simulink model "ACC_test_sim"  (R2023a)
settings: Solver=FixedStepAuto  StartTime=0.0  StopTime=100  FixedStep=0.001  RelTol=1e-3
values from neighbouring files (symbols this model uses):
  b = 50    [ACC_test.m]
  den = [m b]    [ACC_test.m]
  den_dc = [1 (1/J)*(D+KtRa*Kb)]    [ACC_test.m]
  m = 1000    [ACC_test.m]
  num = 1    [ACC_test.m]
  num_dc = KtRa/J    (= 4916.66666667)    [ACC_test.m]
undefined symbols (not defined in the file or in its folder): sigbuilder_block
libraries: slpidlib x10, simulink x6, simulink_extras x6, sim3dautolib x6, sim3dlib x3, mpclib x1
(part 1 of 2)
settings Model: Creator=joeri  LastModifiedBy=joeri
settings DataIOCC: ReturnWorkspaceOutputs=off
settings ModelReferenceCC: EnableRefExpFcnMdlSchedulingChecks=on

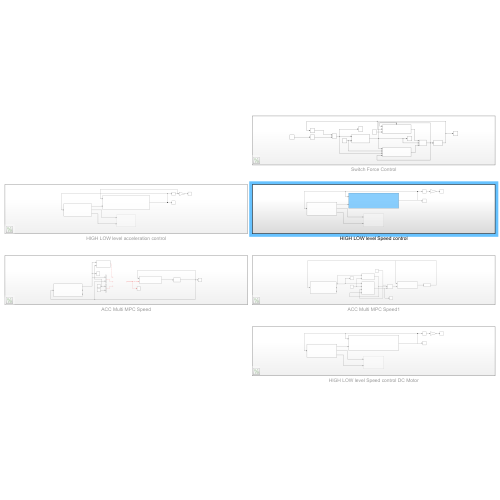
[thumbnail: Simulink's stored preview of the top-level diagram]
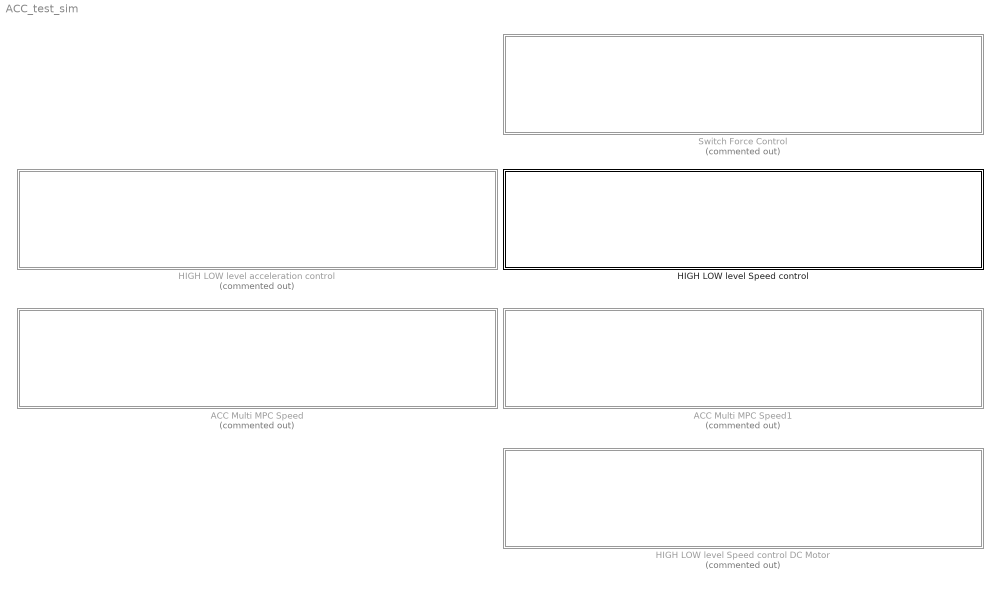
== system ACC_test_sim ==
  ACC Multi MPC Speed : Subsystem  Commented=on
  ACC Multi MPC Speed1 : Subsystem  Commented=on
  HIGH LOW level Speed control : Subsystem
  HIGH LOW level Speed control DC Motor : Subsystem  Commented=on
  HIGH LOW level acceleration control : Subsystem  Commented=on
  Switch Force Control : Subsystem  Commented=on

== system ACC_test_sim/ACC Multi MPC Speed ==
  Constant1 : Constant  Value=30/3.6
  Constant2 : Constant  Value=20
  Mux : Mux  Inputs=2
  Mux1 : Mux  Inputs=2
  Scope : Scope
  Scope1 : Scope
  Scope2 : Scope
  Sensors : Subsystem
  Speed Feedback Control : Subsystem
  Switcher : Subsystem
  Transfer Fcn (with initial outputs) : simulink_extras/Additional Linear/Transfer Fcn (with initial outputs)  N=num  D=den  Y0=30/3.6  U0=0
  wires:
  Transfer Fcn (with initial outputs)/1 -> Speed Feedback Control/1(Reference speed), Scope/1, Mux1/2, Sensors/1(MORE Vehicle speed)  "MORE Vehicle Speed"
  Speed Feedback Control/1(Control effort) -> Transfer Fcn (with initial outputs)/1
  ? -> Scope2/1, Speed Feedback Control/2(Speed)
  Sensors/1(Distance Gap) -> Switcher/1(Gap), Scope1/1, Mux1/1
  Constant1/1 -> Mux/2
  Constant2/1 -> Switcher/2(Desired Distance), Mux/1
  Mux/1 -> ?
  Mux1/1 -> ?
  Switcher/1(Output) -> ?

== system ACC_test_sim/ACC Multi MPC Speed1 ==
  Constant : Constant  Value=20
  MPC Speed : mpclib/MPC Controller  SCDEnableBlockLinearizationSpecification=on  mpcobj=mpc1  is_multiple=0  enable_value=0  return_u0=off  updateMPCinCallerWorkspace=on  md_inport=off  mv_inport=off  uref_inport=off  return_cost=off  return_mvseq=off  return_qpstatus=off  return_xseq=off  return_state=off  return_ovseq=off  state_inport=off  umin_inport=off  umax_inport=off  ymin_inport=off  ymax_inport=on  cc_inport=off  ywt_inport=off  uwt_inport=off  duwt_inport=off  rhoeps_inport=off  pm_inport=off  MaximumP=10  HorizonChoice=FixedHorizon  n_ts=0.1  n_p=30  n_mv=1  n_md=0  n_ud=0  n_mo=1  n_uo=0  BlockDataType=double  SampleTimeInherited=off  switch_inport=on
  Scope1 : Scope
  Scope2 : Scope
  Sensors : Subsystem
  Speed Feedback Control : Subsystem
  Switch : Switch  Criteria=u2 > Threshold  SaturateOnIntegerOverflow=off  InputSameDT=off
  Switcher : Subsystem
  Transfer Fcn (with initial outputs) : simulink_extras/Additional Linear/Transfer Fcn (with initial outputs)  N=num  D=den  Y0=30/3.6  U0=0
  v_d : Constant  Value=30/3.6
  wires:
  Transfer Fcn (with initial outputs)/1 -> Sensors/1(MORE Vehicle speed), Speed Feedback Control/1(Reference speed)  "MORE Vehicle Speed"
  Sensors/1(Distance Gap) -> Switcher/1(Gap), Scope1/1, MPC Speed/1
  Speed Feedback Control/1(Control effort) -> Transfer Fcn (with initial outputs)/1
  Constant/1 -> MPC Speed/2, Switcher/2(Desired Distance)
  Switch/1 -> Speed Feedback Control/2(Speed setpoint)
  MPC Speed/1 -> Scope2/1, Switch/3
  v_d/1 -> MPC Speed/3, Switch/1
  Switcher/1(Output) -> MPC Speed/4, Switch/2

== system ACC_test_sim/HIGH LOW level Speed control ==
  3D Sim : Subsystem  Commented=on
  Derivative : Derivative
  Model And Control : Subsystem
  Scope1 : Scope
  Scope2 : Scope
  Sensors : Subsystem
  m/s/s to G : Gain  Gain=1/9.81
  wires:
  Derivative/1 -> m/s/s to G/1
  m/s/s to G/1 -> Scope2/1
  Model And Control/1(MORE Vehicle Speed [m/s]) -> Scope1/1, Model And Control/1(Reference speed [m/s]), Sensors/1(MORE Vehicle speed), Derivative/1
  Sensors/1(Distance Gap) -> Model And Control/2(Distance Gap [m])
  Sensors/2(MORE Vehicle distance) -> 3D Sim/1(MORE Vehicle Distance)
  Sensors/3(Leading Vehicle distance) -> 3D Sim/2(Leading Vehicle distance)

== system ACC_test_sim/HIGH LOW level Speed control DC Motor ==
  3D Sim : Subsystem  Commented=on
  Derivative : Derivative
  Model And Control : Subsystem
  Scope1 : Scope
  Scope2 : Scope
  Sensors : Subsystem
  m/s/s to G : Gain  Gain=1/9.81
  wires:
  Derivative/1 -> m/s/s to G/1
  m/s/s to G/1 -> Scope2/1
  Model And Control/1(MORE Vehicle Speed) -> Scope1/1, Model And Control/1(Reference speed), Sensors/1(MORE Vehicle speed), Derivative/1
  Sensors/1(Distance Gap) -> Model And Control/2(Distance Gap)
  Sensors/2(MORE Vehicle distance) -> 3D Sim/1(MORE Vehicle Distance)
  Sensors/3(Leading Vehicle distance) -> 3D Sim/2(Leading Vehicle distance)

== system ACC_test_sim/HIGH LOW level acceleration control ==
  3D Sim : Subsystem  Commented=on
  Derivative : Derivative
  Model And Control : Subsystem
  Scope1 : Scope
  Scope2 : Scope
  Sensors : Subsystem
  m/s/s to G : Gain  Gain=1/9.81
  wires:
  Derivative/1 -> Model And Control/1(Reference acc.), m/s/s to G/1
  m/s/s to G/1 -> Scope2/1
  Model And Control/1(MORE Vehicle Speed) -> Scope1/1, Sensors/1(MORE Vehicle speed), Derivative/1
  Sensors/1(Distance Gap) -> Model And Control/2(Distance Gap)
  Sensors/2(MORE Vehicle distance) -> 3D Sim/1(MORE Vehicle Distance)
  Sensors/3(Leading Vehicle distance) -> 3D Sim/2(Leading Vehicle distance)

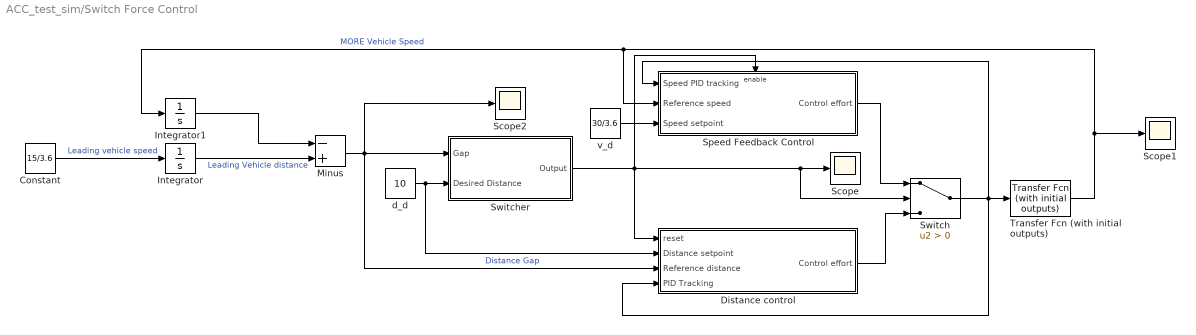
== system ACC_test_sim/Switch Force Control ==
  Constant : Constant  Value=15/3.6
  Distance control : Subsystem
  Integrator : Integrator  InitialCondition=100
  Integrator1 : Integrator
  Minus : Sum  Inputs=-+
  Scope : Scope
  Scope1 : Scope
  Scope2 : Scope
  Speed Feedback Control : Subsystem
  Switch : Switch  Criteria=u2 > Threshold  SaturateOnIntegerOverflow=off  InputSameDT=off
  Switcher : Subsystem
  Transfer Fcn (with initial outputs) : simulink_extras/Additional Linear/Transfer Fcn (with initial outputs)  N=num  D=den  Y0=30/3.6  U0=0
  d_d : Constant  Value=10
  v_d : Constant  Value=30/3.6
  wires:
  Minus/1 -> Switcher/1(Gap), Scope2/1, Distance control/3(Reference distance)  "Distance Gap"
  Distance control/1(Control effort) -> Switch/3
  Speed Feedback Control/1(Control effort) -> Switch/1
  Transfer Fcn (with initial outputs)/1 -> Speed Feedback Control/2(Reference speed), Integrator1/1, Scope1/1  "MORE Vehicle Speed"
  Switch/1 -> Speed Feedback Control/1(Speed PID tracking), Distance control/4(PID Tracking), Transfer Fcn (with initial outputs)/1
  Switcher/1(Output) -> Speed Feedback Control/Enable, Distance control/1(reset), Scope/1, Switch/2
  Integrator/1 -> Minus/2  "Leading Vehicle distance"
  v_d/1 -> Speed Feedback Control/3(Speed setpoint)
  d_d/1 -> Distance control/2(Distance setpoint), Switcher/2(Desired Distance)
  Integrator1/1 -> Minus/1
  Constant/1 -> Integrator/1  "Leading vehicle speed"

== system ACC_test_sim/ACC Multi MPC Speed/Sensors ==
  MORE Vehicle speed : Inport
  Constant : Constant  Value=20/3.6
  Integrator : Integrator  InitialCondition=100
  Integrator1 : Integrator
  Minus : Sum  Inputs=-+
  Minus1 : Sum  Inputs=+-
  Signal Builder : Subsystem  Tag=STV Subsys  LoadFcn=sigbuilder_block('load');  StartFcn=sigbuilder_block('start');  StopFcn=sigbuilder_block('stop');  ClipboardFcn=sigbuilder_block('clipboard');  mask(Sigbuilder block){tuvar=[0:10]}
      mask help: Simulink:masks:SigbuilderBlock_MD
      mask init:
      | if ~strcmp(get_param(bdroot(gcbh),'SimulationStatus'),'stopped') tuvar = sigbuilder_block('maskInit'); end
      settings: CopyFcn=sigbuilder_block('copy');  DeleteFcn=sigbuilder_block('delete');  ModelCloseFcn=sigbuilder_block('modelClose');  PreSaveFcn=sigbuilder_block('preSave');  PauseFcn=sigbuilder_block('pause');  ContinueFcn=sigbuilder_block('continue');  NameChangeFcn=sigbuilder_block('namechange');  OpenFcn=sigbuilder_block('open',[446.4 127.8 550.8 400.2 ]);  CloseFcn=sigbuilder_block('close');
      mask Display: plot(0, 0, 100, 100,[2, 2, 32, 32, 2], [68, 8, 8, 68, 68],[32, 2], [38, 38], [32, 19, 2],[53, 60, 44], [32, 17, 17, 2],[16, 16, 31, 31]);txt = getActiveGroup(gcbh);text(2, 100, txt,'verticalAlignment', 'top');
  Distance Gap : Outport
  MORE Vehicle distance : Outport  Port=2
  Relative speed : Outport  Port=3
  wires:
  Constant/1 -> Integrator/1, Minus1/2  "Leading vehicle speed"
  Minus1/1 -> Relative speed/1
  Minus/1 -> Distance Gap/1  "Distance Gap"
  Integrator1/1 -> MORE Vehicle distance/1, Minus/1
  MORE Vehicle speed/1 -> Integrator1/1, Minus1/1
  Integrator/1 -> Minus/2  "Leading Vehicle distance"

== system ACC_test_sim/ACC Multi MPC Speed/Speed Feedback Control ==
  Reference speed : Inport
  Speed : Inport  Port=2
  -5000 -5000 N1 : Saturate  UpperLimit=5000  LowerLimit=-5000
  Add : Sum
  Feed Forward : Subsystem
  PID Controller : slpidlib/PID Controller  Controller=PID  Form=Parallel  TimeDomain=Continuous-time  UseExternalTs=off  SampleTime=-1  IntegratorMethod=Forward Euler  FilterMethod=Forward Euler  ControllerParametersSource=internal  P=2000  I=50  UseKiTs=off  D=10  N=100  UseFilter=on  TunerSelectOption=Transfer Function Based (PID Tuner App)  InitialConditionSource=internal  InitialConditionForIntegrator=0  InitialConditionForFilter=0  DifferentiatorICPrevScaledInput=0  ExternalReset=none  TrackingMode=off  Kt=0  LimitOutput=on  SatLimitsSource=internal  UpperSaturationLimit=5000  LowerSaturationLimit=-5000  LinearizeAsGain=on  AntiWindupMode=clamping  Kb=1  POutMin=[]  POutMax=[]  IOutMin=[]  IOutMax=[]  DOutMin=[]  DOutMax=[]  NOutMin=[]  NOutMax=[]  SumOutMin=[]  SumOutMax=[]  SaturationOutMin=[]  SaturationOutMax=[]  PParamMin=[]  PParamMax=[]  IParamMin=[]  IParamMax=[]  DParamMin=[]  DParamMax=[]  NParamMin=[]  NParamMax=[]  KbParamMin=[]  KbParamMax=[]  KtParamMin=[]  KtParamMax=[]  KbOutMin=[]  KbOutMax=[]  KtOutMin=[]  KtOutMax=[]  IntegratorOutMin=[]  IntegratorOutMax=[]  FilterOutMin=[]  FilterOutMax=[]  SumI1OutMin=[]  SumI1OutMax=[]  SumI2OutMin=[]  SumI2OutMax=[]  SumI3OutMin=[]  SumI3OutMax=[]  SumI4OutMin=[]  SumI4OutMax=[]  SumDOutMin=[]  SumDOutMax=[]  DifferentiatorOutMin=[]  DifferentiatorOutMax=[]  FilterDiffOutCoefMin=[]  FilterDiffOutCoefMax=[]  ReciprocalOutMin=[]  ReciprocalOutMax=[]  SumDenOutMin=[]  SumDenOutMax=[]  SumNumOutMin=[]  SumNumOutMax=[]  DivideOutMin=[]  DivideOutMax=[]  UdiffTsProdOutMin=[]  UdiffTsProdOutMax=[]  NTsProdOutMin=[]  NTsProdOutMax=[]  UintegralTsProdOutMin=[]  UintegralTsProdOutMax=[]  UngainTsProdOutMin=[]  UngainTsProdOutMax=[]  IntegratorContinuousStateAttributes=''  IntegratorStateMustResolveToSignalObject=off  IntegratorRTWStateStorageClass=Auto  FilterContinuousStateAttributes=''  FilterStateMustResolveToSignalObject=off  FilterRTWStateStorageClass=Auto  ParallelPVariant=InternalParameters  IdealPVariant=Disabled  IVariant=InternalParameters  DVariant=InternalParameters  IntegratorVariant=Continuous  SatVariant=Enabled  AWVariant=ContClampingParallel  PCopyVariant=Disabled  TRVariant=Disabled  FdbkBlocksVariant=Forward  IdealPFdbkVariant=Disabled  SatFdbkVariant=Disabled  DerivativeFilterVariant=ContFilter  NVariant=InternalParameters  NCopyVariant=Disabled  FilterICVariant=InternalICsFilter  IntegratorICVariant=InternalICs  ExternalResetVariant=Disabled  TRSumVariant=Passthrough  SumFdbkVariant=Disabled  SumVariant=Sum_PID  TsampFilterVariant=InternalTs  TsampNgainVariant=Passthrough  TsampIntegralVariant=Passthrough  ExternalSaturationOutDataTypeStr=Inherit: Same as second input  aMode=0
  Scope : Scope  NumInputPorts=3
  Sum1 : Sum  Inputs=|+-
  Control effort : Outport
  wires:
  Feed Forward/1(Out1) -> Add/1
  Reference speed/1 -> Sum1/2
  PID Controller/1 -> Add/2, Scope/2  "Controller Output, Force"
  Add/1 -> -5000 -5000 N1/1
  -5000 -5000 N1/1 -> Scope/3, Control effort/1  "Force"
  Speed/1 -> Sum1/1, Feed Forward/1(desired speed1), Scope/1
  Sum1/1 -> PID Controller/1  "E"

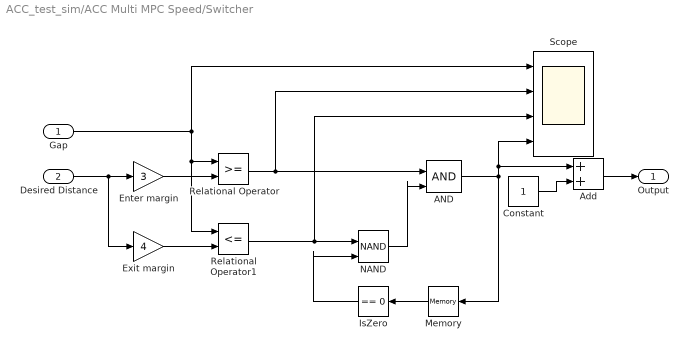
== system ACC_test_sim/ACC Multi MPC Speed/Switcher ==
  Gap : Inport
  Desired Distance : Inport  Port=2
  AND : Logic  IconShape=distinctive  AllPortsSameDT=off  OutDataTypeStr=boolean
  Add : Sum
  Constant : Constant
  Enter margin : Gain  Gain=3
  Exit margin : Gain  Gain=4
  IsZero : simulink/Logic and Bit Operations/Compare To Zero  relop===  OutDataTypeStr=boolean
  Memory : Memory
  NAND : Logic  Operator=NAND  IconShape=distinctive  AllPortsSameDT=off  OutDataTypeStr=boolean
  Relational Operator : RelationalOperator  OutDataTypeStr=boolean  RndMeth=Simplest  InputSameDT=off
  Relational Operator1 : RelationalOperator  Operator=<=  OutDataTypeStr=boolean  RndMeth=Simplest  InputSameDT=off
  Scope : Scope  NumInputPorts=4
  Output : Outport
  wires:
  Enter margin/1 -> Relational Operator/2
  Desired Distance/1 -> Exit margin/1, Enter margin/1
  Exit margin/1 -> Relational Operator1/2
  Relational Operator/1 -> AND/1, Scope/2
  Relational Operator1/1 -> NAND/1, Scope/3
  Memory/1 -> IsZero/1
  NAND/1 -> AND/2
  AND/1 -> Add/1, Scope/4, Memory/1
  IsZero/1 -> NAND/2
  Gap/1 -> Scope/1, Relational Operator1/1, Relational Operator/1
  Add/1 -> Output/1
  Constant/1 -> Add/2

== system ACC_test_sim/ACC Multi MPC Speed1/Sensors ==
  MORE Vehicle speed : Inport
  Constant : Constant  Value=20/3.6
  Integrator : Integrator  InitialCondition=100
  Integrator1 : Integrator
  Minus : Sum  Inputs=-+
  Signal Builder : Subsystem  Tag=STV Subsys  LoadFcn=sigbuilder_block('load');  StartFcn=sigbuilder_block('start');  StopFcn=sigbuilder_block('stop');  ClipboardFcn=sigbuilder_block('clipboard');  mask(Sigbuilder block){tuvar=[0:10]}
      mask help: Simulink:masks:SigbuilderBlock_MD
      mask init:
      | if ~strcmp(get_param(bdroot(gcbh),'SimulationStatus'),'stopped') tuvar = sigbuilder_block('maskInit'); end
      settings: CopyFcn=sigbuilder_block('copy');  DeleteFcn=sigbuilder_block('delete');  ModelCloseFcn=sigbuilder_block('modelClose');  PreSaveFcn=sigbuilder_block('preSave');  PauseFcn=sigbuilder_block('pause');  ContinueFcn=sigbuilder_block('continue');  NameChangeFcn=sigbuilder_block('namechange');  OpenFcn=sigbuilder_block('open',[446.4 127.8 550.8 400.2 ]);  CloseFcn=sigbuilder_block('close');
      mask Display: plot(0, 0, 100, 100,[2, 2, 32, 32, 2], [68, 8, 8, 68, 68],[32, 2], [38, 38], [32, 19, 2],[53, 60, 44], [32, 17, 17, 2],[16, 16, 31, 31]);txt = getActiveGroup(gcbh);text(2, 100, txt,'verticalAlignment', 'top');
  Distance Gap : Outport
  MORE Vehicle distance : Outport  Port=2
  Leading Vehicle distance : Outport  Port=3
  wires:
  Integrator/1 -> Leading Vehicle distance/1, Minus/2  "Leading Vehicle distance"
  MORE Vehicle speed/1 -> Integrator1/1
  Integrator1/1 -> Minus/1, MORE Vehicle distance/1
  Minus/1 -> Distance Gap/1  "Distance Gap"
  Signal Builder/1(Signal 1) -> Integrator/1

== system ACC_test_sim/ACC Multi MPC Speed1/Speed Feedback Control ==
  Reference speed : Inport
  Speed setpoint : Inport  Port=2
  -5000 -5000 N1 : Saturate  UpperLimit=5000  LowerLimit=-5000
  Add : Sum
  Feed Forward : Subsystem
  PID Controller : slpidlib/PID Controller  Controller=PID  Form=Parallel  TimeDomain=Continuous-time  UseExternalTs=off  SampleTime=-1  IntegratorMethod=Forward Euler  FilterMethod=Forward Euler  ControllerParametersSource=internal  P=2000  I=50  UseKiTs=off  D=10  N=100  UseFilter=on  TunerSelectOption=Transfer Function Based (PID Tuner App)  InitialConditionSource=internal  InitialConditionForIntegrator=0  InitialConditionForFilter=0  DifferentiatorICPrevScaledInput=0  ExternalReset=none  TrackingMode=off  Kt=0  LimitOutput=on  SatLimitsSource=internal  UpperSaturationLimit=5000  LowerSaturationLimit=-5000  LinearizeAsGain=on  AntiWindupMode=clamping  Kb=1  POutMin=[]  POutMax=[]  IOutMin=[]  IOutMax=[]  DOutMin=[]  DOutMax=[]  NOutMin=[]  NOutMax=[]  SumOutMin=[]  SumOutMax=[]  SaturationOutMin=[]  SaturationOutMax=[]  PParamMin=[]  PParamMax=[]  IParamMin=[]  IParamMax=[]  DParamMin=[]  DParamMax=[]  NParamMin=[]  NParamMax=[]  KbParamMin=[]  KbParamMax=[]  KtParamMin=[]  KtParamMax=[]  KbOutMin=[]  KbOutMax=[]  KtOutMin=[]  KtOutMax=[]  IntegratorOutMin=[]  IntegratorOutMax=[]  FilterOutMin=[]  FilterOutMax=[]  SumI1OutMin=[]  SumI1OutMax=[]  SumI2OutMin=[]  SumI2OutMax=[]  SumI3OutMin=[]  SumI3OutMax=[]  SumI4OutMin=[]  SumI4OutMax=[]  SumDOutMin=[]  SumDOutMax=[]  DifferentiatorOutMin=[]  DifferentiatorOutMax=[]  FilterDiffOutCoefMin=[]  FilterDiffOutCoefMax=[]  ReciprocalOutMin=[]  ReciprocalOutMax=[]  SumDenOutMin=[]  SumDenOutMax=[]  SumNumOutMin=[]  SumNumOutMax=[]  DivideOutMin=[]  DivideOutMax=[]  UdiffTsProdOutMin=[]  UdiffTsProdOutMax=[]  NTsProdOutMin=[]  NTsProdOutMax=[]  UintegralTsProdOutMin=[]  UintegralTsProdOutMax=[]  UngainTsProdOutMin=[]  UngainTsProdOutMax=[]  IntegratorContinuousStateAttributes=''  IntegratorStateMustResolveToSignalObject=off  IntegratorRTWStateStorageClass=Auto  FilterContinuousStateAttributes=''  FilterStateMustResolveToSignalObject=off  FilterRTWStateStorageClass=Auto  ParallelPVariant=InternalParameters  IdealPVariant=Disabled  IVariant=InternalParameters  DVariant=InternalParameters  IntegratorVariant=Continuous  SatVariant=Enabled  AWVariant=ContClampingParallel  PCopyVariant=Disabled  TRVariant=Disabled  FdbkBlocksVariant=Forward  IdealPFdbkVariant=Disabled  SatFdbkVariant=Disabled  DerivativeFilterVariant=ContFilter  NVariant=InternalParameters  NCopyVariant=Disabled  FilterICVariant=InternalICsFilter  IntegratorICVariant=InternalICs  ExternalResetVariant=Disabled  TRSumVariant=Passthrough  SumFdbkVariant=Disabled  SumVariant=Sum_PID  TsampFilterVariant=InternalTs  TsampNgainVariant=Passthrough  TsampIntegralVariant=Passthrough  ExternalSaturationOutDataTypeStr=Inherit: Same as second input  aMode=0
  Scope : Scope  NumInputPorts=3
  Sum1 : Sum  Inputs=|+-
  Control effort : Outport
  wires:
  Sum1/1 -> PID Controller/1  "E"
  Speed setpoint/1 -> Feed Forward/1(desired speed1), Sum1/1
  -5000 -5000 N1/1 -> Control effort/1, Scope/3  "Force"
  Add/1 -> -5000 -5000 N1/1
  Feed Forward/1(Out1) -> Scope/1, Add/1
  PID Controller/1 -> Scope/2, Add/2  "Controller Output, Force"
  Reference speed/1 -> Sum1/2

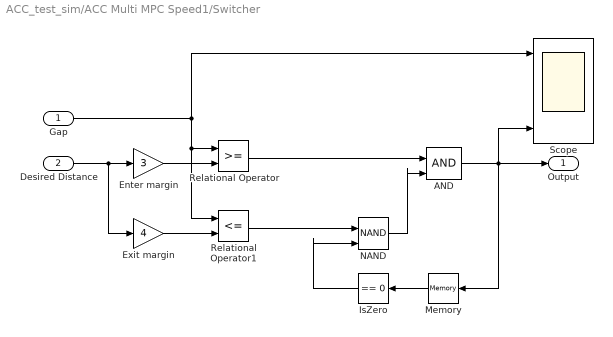
== system ACC_test_sim/ACC Multi MPC Speed1/Switcher ==
  Gap : Inport
  Desired Distance : Inport  Port=2
  AND : Logic  IconShape=distinctive  AllPortsSameDT=off  OutDataTypeStr=boolean
  Enter margin : Gain  Gain=3
  Exit margin : Gain  Gain=4
  IsZero : simulink/Logic and Bit Operations/Compare To Zero  relop===  OutDataTypeStr=boolean
  Memory : Memory
  NAND : Logic  Operator=NAND  IconShape=distinctive  AllPortsSameDT=off  OutDataTypeStr=boolean
  Relational Operator : RelationalOperator  OutDataTypeStr=boolean  RndMeth=Simplest  InputSameDT=off
  Relational Operator1 : RelationalOperator  Operator=<=  OutDataTypeStr=boolean  RndMeth=Simplest  InputSameDT=off
  Scope : Scope  NumInputPorts=4
  Output : Outport
  wires:
  Enter margin/1 -> Relational Operator/2
  Desired Distance/1 -> Exit margin/1, Enter margin/1
  Exit margin/1 -> Relational Operator1/2
  Relational Operator/1 -> AND/1
  Relational Operator1/1 -> NAND/1
  Memory/1 -> IsZero/1
  NAND/1 -> AND/2
  AND/1 -> Scope/4, Memory/1, Output/1
  IsZero/1 -> NAND/2
  Gap/1 -> Scope/1, Relational Operator1/1, Relational Operator/1

== system ACC_test_sim/HIGH LOW level Speed control/3D Sim ==
  MORE Vehicle Distance : Inport
  Leading Vehicle distance : Inport  Port=2
  Constant1 : Constant  Value=0
  Constant2 : Constant  Value=0
  Simulation 3D Scene Configuration : sim3dlib/Simulation 3D Scene Configuration  Priority=0  ProjectFormat=Default Scenes  SceneDesc=Straight road  ProjectName=C:\Program Files\MATLAB\R2022a\toolbox\shared\sim3d_projects\automotive_project\UE4\WindowsNoEditor\VehicleSimulation.exe  ScenePath=/Game/Maps/HwStrght  vehTagList={'Lead';'MORE';'Scene Origin'}  vehTag=MORE  OpVisEn=off  Ts=0.1  EnableWindow=on  EnableRemoteAccess=off  EnableWeather=off  SunAltitude=40.0  SunAzimuth=90  clouds=10  wind=1  fog=0  rain=0  sensorTag=MainCamera1  sensorId=1  sensorName=MainCamera1  mountLoc=Origin  offsetFlag=off  tmountOffset=[0, 0, 0]  rmountOffset=[0, 0, 0]  HorizontalResolution=1280  VerticalResolution=720  HorizontalFOV=60  mountPoint=[0 0 0]  mountOrientation=[0 0 0]  aMode=3  ID=1
  Simulation 3D Vehicle with Ground Following : sim3dautolib/Simulation 3D Vehicle with Ground Following  Priority=-1  PassVehMesh=Muscle car  MeshPath=/MathWorksSimulation/Vehicles/Muscle/Meshes/SK_MuscleCar.SK_MuscleCar  TrackWidth=1.9  WheelBase=3  WheelRadius=0.35  VehColor=Red  InitialPos=[0, 0, 0]  InitialRot=[0, 0, 0]  ActorName=Lead  SampleTime=-1  ActorType=SimulinkVehicle  ID=C  aMode=3  ActorTag=Lead  CoordinateScheme=ISO  VehLightsControl=off  HeadlightColor=[ 1, 1, 1 ]  HighBeamIntensity=100000  LowBeamIntensity=60000  HighBeamConeAngle=70  LowBeamConeAngle=70  LeftHeadlightOrientation=[ 0, 0 ]  RightHeadlightOrientation=[ 0, 0 ]  BrakelightIntensity=500  ReverselightIntensity=500  SignallightIntensity=500  SignallightPeriod=1  SignalPulseWidth=50  TransformOutportEnabled=off
  Simulation 3D Vehicle with Ground Following1 : sim3dautolib/Simulation 3D Vehicle with Ground Following  Priority=-1  PassVehMesh=Muscle car  MeshPath=/MathWorksSimulation/Vehicles/Muscle/Meshes/SK_MuscleCar.SK_MuscleCar  TrackWidth=1.9  WheelBase=3  WheelRadius=0.35  VehColor=Red  InitialPos=[0, 0, 0]  InitialRot=[0, 0, 0]  ActorName=MORE  SampleTime=-1  ActorType=SimulinkVehicle  ID=C  aMode=3  ActorTag=MORE  CoordinateScheme=ISO  VehLightsControl=off  HeadlightColor=[ 1, 1, 1 ]  HighBeamIntensity=100000  LowBeamIntensity=60000  HighBeamConeAngle=70  LowBeamConeAngle=70  LeftHeadlightOrientation=[ 0, 0 ]  RightHeadlightOrientation=[ 0, 0 ]  BrakelightIntensity=500  ReverselightIntensity=500  SignallightIntensity=500  SignallightPeriod=1  SignalPulseWidth=50  TransformOutportEnabled=off
  wires:
  Constant1/1 -> Simulation 3D Vehicle with Ground Following1/2, Simulation 3D Vehicle with Ground Following/2
  Constant2/1 -> Simulation 3D Vehicle with Ground Following/3, Simulation 3D Vehicle with Ground Following1/3
  MORE Vehicle Distance/1 -> Simulation 3D Vehicle with Ground Following1/1
  Leading Vehicle distance/1 -> Simulation 3D Vehicle with Ground Following/1

== system ACC_test_sim/HIGH LOW level Speed control/Model And Control ==
  Reference speed [m/s] : Inport
  Distance Gap [m] : Inport  Port=2
  ACC Distance Control : Subsystem
  CC Speed Feedback Control : Subsystem
  Desired Distance [m] : Constant  Value=20
  Desired Speed [m/s] : Constant  Value=10/3.6
  MORE Vehicle Transfer Function : simulink_extras/Additional Linear/Transfer Fcn (with initial outputs)  N=num  D=den  Y0=30/3.6  U0=0
  Switch : Switch  Criteria=u2 > Threshold  SaturateOnIntegerOverflow=off  InputSameDT=off
  Switcher : Subsystem
  To Workspace : ToWorkspace  VariableName=gap  SampleTime=-1
      settings: Save2DSignal=2-D array (concatenate along first dimension)
  MORE Vehicle Speed [m/s] : Outport
  wires:
  Desired Speed [m/s]/1 -> Switch/1, ACC Distance Control/1(Upper limit)
  Switcher/1(CC to ACC switch) -> Switch/2
  MORE Vehicle Transfer Function/1 -> MORE Vehicle Speed [m/s]/1  "MORE Vehicle Speed"
  ACC Distance Control/1(Speed Setpoint) -> Switch/3
  Distance Gap [m]/1 -> Switcher/1(Gap), To Workspace/1, ACC Distance Control/3(Distance gap)
  CC Speed Feedback Control/1(Control Effort [N]) -> MORE Vehicle Transfer Function/1
  Switch/1 -> ACC Distance Control/4(PID Tracking), CC Speed Feedback Control/2(Speed setpoint [m/s])
  Desired Distance [m]/1 -> ACC Distance Control/2(Distance setpoint), Switcher/2(Desired Distance)
  Reference speed [m/s]/1 -> CC Speed Feedback Control/1(Reference speed [m/s])

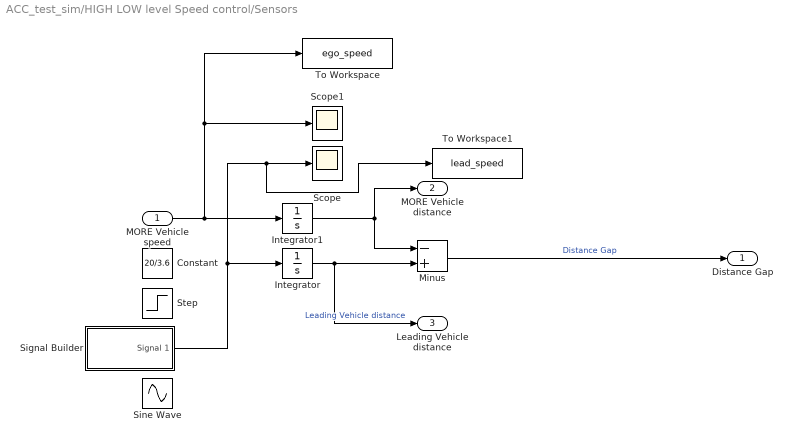
== system ACC_test_sim/HIGH LOW level Speed control/Sensors ==
  MORE Vehicle speed : Inport
  Constant : Constant  Value=20/3.6
  Integrator : Integrator  InitialCondition=100
  Integrator1 : Integrator
  Minus : Sum  Inputs=-+
  Scope : Scope
  Scope1 : Scope
  Signal Builder : Subsystem  Tag=STV Subsys  LoadFcn=sigbuilder_block('load');  StartFcn=sigbuilder_block('start');  StopFcn=sigbuilder_block('stop');  ClipboardFcn=sigbuilder_block('clipboard');  mask(Sigbuilder block){tuvar=[0:10]}
      mask help: Simulink:masks:SigbuilderBlock_MD
      mask init:
      | if ~strcmp(get_param(bdroot(gcbh),'SimulationStatus'),'stopped') tuvar = sigbuilder_block('maskInit'); end
      settings: CopyFcn=sigbuilder_block('copy');  DeleteFcn=sigbuilder_block('delete');  ModelCloseFcn=sigbuilder_block('modelClose');  PreSaveFcn=sigbuilder_block('preSave');  PauseFcn=sigbuilder_block('pause');  ContinueFcn=sigbuilder_block('continue');  NameChangeFcn=sigbuilder_block('namechange');  OpenFcn=sigbuilder_block('open',[446.4 127.8 550.8 400.2 ]);  CloseFcn=sigbuilder_block('close');
      mask Display: plot(0, 0, 100, 100,[2, 2, 32, 32, 2], [68, 8, 8, 68, 68],[32, 2], [38, 38], [32, 19, 2],[53, 60, 44], [32, 17, 17, 2],[16, 16, 31, 31]);txt = getActiveGroup(gcbh);text(2, 100, txt,'verticalAlignment', 'top');
  Sine Wave : Sin  Amplitude=3  Bias=15/3.6  Frequency=0.3  SampleTime=0
  Step : Step  Time=70  Before=20/3.6  After=10/3.6  SampleTime=0
  To Workspace : ToWorkspace  VariableName=ego_speed  SampleTime=-1
      settings: Save2DSignal=2-D array (concatenate along first dimension)
  To Workspace1 : ToWorkspace  VariableName=lead_speed  SampleTime=-1
      settings: Save2DSignal=2-D array (concatenate along first dimension)
  Distance Gap : Outport
  MORE Vehicle distance : Outport  Port=2
  Leading Vehicle distance : Outport  Port=3
  wires:
  Integrator/1 -> Leading Vehicle distance/1, Minus/2  "Leading Vehicle distance"
  MORE Vehicle speed/1 -> To Workspace/1, Scope1/1, Integrator1/1
  Integrator1/1 -> Minus/1, MORE Vehicle distance/1
  Minus/1 -> Distance Gap/1  "Distance Gap"
  Signal Builder/1(Signal 1) -> To Workspace1/1, Scope/1, Integrator/1

== system ACC_test_sim/HIGH LOW level Speed control DC Motor/3D Sim ==
  MORE Vehicle Distance : Inport
  Leading Vehicle distance : Inport  Port=2
  Constant1 : Constant  Value=0
  Constant2 : Constant  Value=0
  Simulation 3D Scene Configuration : sim3dlib/Simulation 3D Scene Configuration  Priority=0  ProjectFormat=Default Scenes  SceneDesc=Straight road  ProjectName=C:\Program Files\MATLAB\R2022a\toolbox\shared\sim3d_projects\automotive_project\UE4\WindowsNoEditor\VehicleSimulation.exe  ScenePath=/Game/Maps/HwStrght  vehTagList={'Lead';'MORE';'Scene Origin'}  vehTag=MORE  OpVisEn=off  Ts=0.1  EnableWindow=on  EnableRemoteAccess=off  EnableWeather=off  SunAltitude=40.0  SunAzimuth=90  clouds=10  wind=1  fog=0  rain=0  sensorTag=MainCamera1  sensorId=1  sensorName=MainCamera1  mountLoc=Origin  offsetFlag=off  tmountOffset=[0, 0, 0]  rmountOffset=[0, 0, 0]  HorizontalResolution=1280  VerticalResolution=720  HorizontalFOV=60  mountPoint=[0 0 0]  mountOrientation=[0 0 0]  aMode=3  ID=1
  Simulation 3D Vehicle with Ground Following : sim3dautolib/Simulation 3D Vehicle with Ground Following  Priority=-1  PassVehMesh=Muscle car  MeshPath=/MathWorksSimulation/Vehicles/Muscle/Meshes/SK_MuscleCar.SK_MuscleCar  TrackWidth=1.9  WheelBase=3  WheelRadius=0.35  VehColor=Red  InitialPos=[0, 0, 0]  InitialRot=[0, 0, 0]  ActorName=Lead  SampleTime=-1  ActorType=SimulinkVehicle  ID=C  aMode=3  ActorTag=Lead  CoordinateScheme=ISO  VehLightsControl=off  HeadlightColor=[ 1, 1, 1 ]  HighBeamIntensity=100000  LowBeamIntensity=60000  HighBeamConeAngle=70  LowBeamConeAngle=70  LeftHeadlightOrientation=[ 0, 0 ]  RightHeadlightOrientation=[ 0, 0 ]  BrakelightIntensity=500  ReverselightIntensity=500  SignallightIntensity=500  SignallightPeriod=1  SignalPulseWidth=50  TransformOutportEnabled=off
  Simulation 3D Vehicle with Ground Following1 : sim3dautolib/Simulation 3D Vehicle with Ground Following  Priority=-1  PassVehMesh=Muscle car  MeshPath=/MathWorksSimulation/Vehicles/Muscle/Meshes/SK_MuscleCar.SK_MuscleCar  TrackWidth=1.9  WheelBase=3  WheelRadius=0.35  VehColor=Red  InitialPos=[0, 0, 0]  InitialRot=[0, 0, 0]  ActorName=MORE  SampleTime=-1  ActorType=SimulinkVehicle  ID=C  aMode=3  ActorTag=MORE  CoordinateScheme=ISO  VehLightsControl=off  HeadlightColor=[ 1, 1, 1 ]  HighBeamIntensity=100000  LowBeamIntensity=60000  HighBeamConeAngle=70  LowBeamConeAngle=70  LeftHeadlightOrientation=[ 0, 0 ]  RightHeadlightOrientation=[ 0, 0 ]  BrakelightIntensity=500  ReverselightIntensity=500  SignallightIntensity=500  SignallightPeriod=1  SignalPulseWidth=50  TransformOutportEnabled=off
  wires:
  Constant1/1 -> Simulation 3D Vehicle with Ground Following1/2, Simulation 3D Vehicle with Ground Following/2
  Constant2/1 -> Simulation 3D Vehicle with Ground Following/3, Simulation 3D Vehicle with Ground Following1/3
  MORE Vehicle Distance/1 -> Simulation 3D Vehicle with Ground Following1/1
  Leading Vehicle distance/1 -> Simulation 3D Vehicle with Ground Following/1

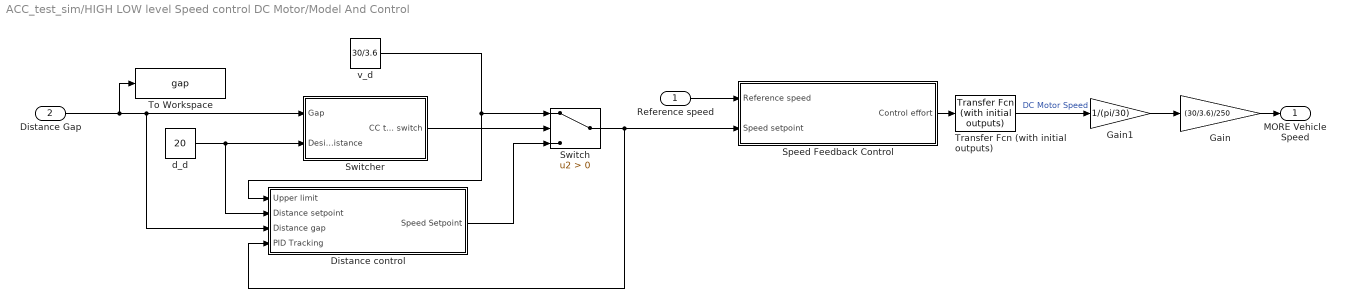
== system ACC_test_sim/HIGH LOW level Speed control DC Motor/Model And Control ==
  Reference speed : Inport
  Distance Gap : Inport  Port=2
  Distance control : Subsystem
  Gain : Gain  Gain=(30/3.6)/250
  Gain1 : Gain  Gain=1/(pi/30)
  Speed Feedback Control : Subsystem
  Switch : Switch  Criteria=u2 > Threshold  SaturateOnIntegerOverflow=off  InputSameDT=off
  Switcher : Subsystem
  To Workspace : ToWorkspace  VariableName=gap  SampleTime=-1
      settings: Save2DSignal=2-D array (concatenate along first dimension)
  Transfer Fcn (with initial outputs) : simulink_extras/Additional Linear/Transfer Fcn (with initial outputs)  N=num_dc  D=den_dc  Y0=250/(pi/30)  U0=0
  d_d : Constant  Value=20
  v_d : Constant  Value=30/3.6
  MORE Vehicle Speed : Outport
  wires:
  v_d/1 -> Switch/1, Distance control/1(Upper limit)
  Switcher/1(CC to ACC switch) -> Switch/2
  Transfer Fcn (with initial outputs)/1 -> Gain1/1  "DC Motor Speed"
  Distance control/1(Speed Setpoint) -> Switch/3
  Distance Gap/1 -> To Workspace/1, Switcher/1(Gap), Distance control/3(Distance gap)
  Speed Feedback Control/1(Control effort) -> Transfer Fcn (with initial outputs)/1
  Switch/1 -> Distance control/4(PID Tracking), Speed Feedback Control/2(Speed setpoint)
  d_d/1 -> Distance control/2(Distance setpoint), Switcher/2(Desired Distance)
  Reference speed/1 -> Speed Feedback Control/1(Reference speed)
  Gain/1 -> MORE Vehicle Speed/1
  Gain1/1 -> Gain/1

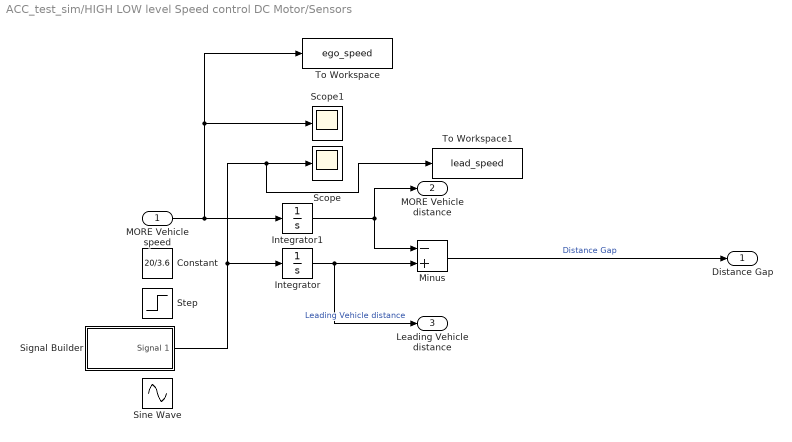
== system ACC_test_sim/HIGH LOW level Speed control DC Motor/Sensors ==
  MORE Vehicle speed : Inport
  Constant : Constant  Value=20/3.6
  Integrator : Integrator  InitialCondition=100
  Integrator1 : Integrator
  Minus : Sum  Inputs=-+
  Scope : Scope
  Scope1 : Scope
  Signal Builder : Subsystem  Tag=STV Subsys  LoadFcn=sigbuilder_block('load');  StartFcn=sigbuilder_block('start');  StopFcn=sigbuilder_block('stop');  ClipboardFcn=sigbuilder_block('clipboard');  mask(Sigbuilder block){tuvar=[0:10]}
      mask help: Simulink:masks:SigbuilderBlock_MD
      mask init:
      | if ~strcmp(get_param(bdroot(gcbh),'SimulationStatus'),'stopped') tuvar = sigbuilder_block('maskInit'); end
      settings: CopyFcn=sigbuilder_block('copy');  DeleteFcn=sigbuilder_block('delete');  ModelCloseFcn=sigbuilder_block('modelClose');  PreSaveFcn=sigbuilder_block('preSave');  PauseFcn=sigbuilder_block('pause');  ContinueFcn=sigbuilder_block('continue');  NameChangeFcn=sigbuilder_block('namechange');  OpenFcn=sigbuilder_block('open',[446.4 127.8 550.8 400.2 ]);  CloseFcn=sigbuilder_block('close');
      mask Display: plot(0, 0, 100, 100,[2, 2, 32, 32, 2], [68, 8, 8, 68, 68],[32, 2], [38, 38], [32, 19, 2],[53, 60, 44], [32, 17, 17, 2],[16, 16, 31, 31]);txt = getActiveGroup(gcbh);text(2, 100, txt,'verticalAlignment', 'top');
  Sine Wave : Sin  Amplitude=3  Bias=15/3.6  Frequency=0.3  SampleTime=0
  Step : Step  Time=70  Before=20/3.6  After=10/3.6  SampleTime=0
  To Workspace : ToWorkspace  VariableName=ego_speed  SampleTime=-1
      settings: Save2DSignal=2-D array (concatenate along first dimension)
  To Workspace1 : ToWorkspace  VariableName=lead_speed  SampleTime=-1
      settings: Save2DSignal=2-D array (concatenate along first dimension)
  Distance Gap : Outport
  MORE Vehicle distance : Outport  Port=2
  Leading Vehicle distance : Outport  Port=3
  wires:
  Integrator/1 -> Leading Vehicle distance/1, Minus/2  "Leading Vehicle distance"
  MORE Vehicle speed/1 -> To Workspace/1, Scope1/1, Integrator1/1
  Integrator1/1 -> Minus/1, MORE Vehicle distance/1
  Minus/1 -> Distance Gap/1  "Distance Gap"
  Signal Builder/1(Signal 1) -> To Workspace1/1, Scope/1, Integrator/1

== system ACC_test_sim/HIGH LOW level acceleration control/3D Sim ==
  MORE Vehicle Distance : Inport
  Leading Vehicle distance : Inport  Port=2
  Constant1 : Constant  Value=0
  Constant2 : Constant  Value=0
  Simulation 3D Scene Configuration : sim3dlib/Simulation 3D Scene Configuration  Priority=0  ProjectFormat=Default Scenes  SceneDesc=Straight road  ProjectName=C:\Program Files\MATLAB\R2022a\toolbox\shared\sim3d_projects\automotive_project\UE4\WindowsNoEditor\VehicleSimulation.exe  ScenePath=/Game/Maps/HwStrght  vehTagList={'Lead';'MORE';'Scene Origin'}  vehTag=MORE  OpVisEn=off  Ts=0.1  EnableWindow=on  EnableRemoteAccess=off  EnableWeather=off  SunAltitude=40.0  SunAzimuth=90  clouds=10  wind=1  fog=0  rain=0  sensorTag=MainCamera2  sensorId=2  sensorName=MainCamera2  mountLoc=Origin  offsetFlag=off  tmountOffset=[0, 0, 0]  rmountOffset=[0, 0, 0]  HorizontalResolution=1280  VerticalResolution=720  HorizontalFOV=60  mountPoint=[0 0 0]  mountOrientation=[0 0 0]  aMode=3  ID=2
  Simulation 3D Vehicle with Ground Following : sim3dautolib/Simulation 3D Vehicle with Ground Following  Priority=-1  PassVehMesh=Muscle car  MeshPath=/MathWorksSimulation/Vehicles/Muscle/Meshes/SK_MuscleCar.SK_MuscleCar  TrackWidth=1.9  WheelBase=3  WheelRadius=0.35  VehColor=Red  InitialPos=[0, 0, 0]  InitialRot=[0, 0, 0]  ActorName=SimulinkVehicle1  SampleTime=-1  ActorType=SimulinkVehicle  ID=1  aMode=3  ActorTag=SimulinkVehicle1  CoordinateScheme=ISO  VehLightsControl=off  HeadlightColor=[ 1, 1, 1 ]  HighBeamIntensity=100000  LowBeamIntensity=60000  HighBeamConeAngle=70  LowBeamConeAngle=70  LeftHeadlightOrientation=[ 0, 0 ]  RightHeadlightOrientation=[ 0, 0 ]  BrakelightIntensity=500  ReverselightIntensity=500  SignallightIntensity=500  SignallightPeriod=1  SignalPulseWidth=50  TransformOutportEnabled=off
  Simulation 3D Vehicle with Ground Following1 : sim3dautolib/Simulation 3D Vehicle with Ground Following  Priority=-1  PassVehMesh=Muscle car  MeshPath=/MathWorksSimulation/Vehicles/Muscle/Meshes/SK_MuscleCar.SK_MuscleCar  TrackWidth=1.9  WheelBase=3  WheelRadius=0.35  VehColor=Red  InitialPos=[0, 0, 0]  InitialRot=[0, 0, 0]  ActorName=SimulinkVehicle2  SampleTime=-1  ActorType=SimulinkVehicle  ID=2  aMode=3  ActorTag=SimulinkVehicle2  CoordinateScheme=ISO  VehLightsControl=off  HeadlightColor=[ 1, 1, 1 ]  HighBeamIntensity=100000  LowBeamIntensity=60000  HighBeamConeAngle=70  LowBeamConeAngle=70  LeftHeadlightOrientation=[ 0, 0 ]  RightHeadlightOrientation=[ 0, 0 ]  BrakelightIntensity=500  ReverselightIntensity=500  SignallightIntensity=500  SignallightPeriod=1  SignalPulseWidth=50  TransformOutportEnabled=off
  wires:
  Constant1/1 -> Simulation 3D Vehicle with Ground Following1/2, Simulation 3D Vehicle with Ground Following/2
  Constant2/1 -> Simulation 3D Vehicle with Ground Following/3, Simulation 3D Vehicle with Ground Following1/3
  MORE Vehicle Distance/1 -> Simulation 3D Vehicle with Ground Following1/1
  Leading Vehicle distance/1 -> Simulation 3D Vehicle with Ground Following/1

== system ACC_test_sim/HIGH LOW level acceleration control/Model And Control ==
  Reference acc. : Inport
  Distance Gap : Inport  Port=2
  Distance control : Subsystem
  Scope : Scope
  Speed Feedback Control : Subsystem
  Switch : Switch  Criteria=u2 > Threshold  SaturateOnIntegerOverflow=off  InputSameDT=off
  Switcher : Subsystem
  Transfer Fcn (with initial outputs) : simulink_extras/Additional Linear/Transfer Fcn (with initial outputs)  N=num  D=den  Y0=30/3.6  U0=0
  d_d : Constant  Value=20
  v_d : Constant  Value=30/3.6
  MORE Vehicle Speed : Outport
  wires:
  v_d/1 -> Switch/1, Distance control/1(Upper limit)
  Switcher/1(Output) -> Switch/2
  Transfer Fcn (with initial outputs)/1 -> MORE Vehicle Speed/1  "MORE Vehicle Speed"
  Distance control/1(Acceleration setpoint) -> Switch/3
  Distance Gap/1 -> Scope/1, Switcher/1(Gap), Distance control/3(Distance gap)
  Speed Feedback Control/1(Control effort) -> Transfer Fcn (with initial outputs)/1
  Switch/1 -> Distance control/4(PID Tracking), Speed Feedback Control/2(Acceleration)
  d_d/1 -> Distance control/2(Distance setpoint), Switcher/2(Desired Distance)
  Reference acc./1 -> Speed Feedback Control/1(Reference acc.)

== system ACC_test_sim/HIGH LOW level acceleration control/Sensors ==
  MORE Vehicle speed : Inport
  Constant : Constant  Value=20/3.6
  Integrator : Integrator  InitialCondition=100
  Integrator1 : Integrator
  Minus : Sum  Inputs=-+
  Signal Builder : Subsystem  Tag=STV Subsys  LoadFcn=sigbuilder_block('load');  StartFcn=sigbuilder_block('start');  StopFcn=sigbuilder_block('stop');  ClipboardFcn=sigbuilder_block('clipboard');  mask(Sigbuilder block){tuvar=[0:10]}
      mask help: Simulink:masks:SigbuilderBlock_MD
      mask init:
      | if ~strcmp(get_param(bdroot(gcbh),'SimulationStatus'),'stopped') tuvar = sigbuilder_block('maskInit'); end
      settings: CopyFcn=sigbuilder_block('copy');  DeleteFcn=sigbuilder_block('delete');  ModelCloseFcn=sigbuilder_block('modelClose');  PreSaveFcn=sigbuilder_block('preSave');  PauseFcn=sigbuilder_block('pause');  ContinueFcn=sigbuilder_block('continue');  NameChangeFcn=sigbuilder_block('namechange');  OpenFcn=sigbuilder_block('open',[446.4 127.8 550.8 400.2 ]);  CloseFcn=sigbuilder_block('close');
      mask Display: plot(0, 0, 100, 100,[2, 2, 32, 32, 2], [68, 8, 8, 68, 68],[32, 2], [38, 38], [32, 19, 2],[53, 60, 44], [32, 17, 17, 2],[16, 16, 31, 31]);txt = getActiveGroup(gcbh);text(2, 100, txt,'verticalAlignment', 'top');
  Distance Gap : Outport
  MORE Vehicle distance : Outport  Port=2
  Leading Vehicle distance : Outport  Port=3
  wires:
  Integrator/1 -> Leading Vehicle distance/1, Minus/2  "Leading Vehicle distance"
  MORE Vehicle speed/1 -> Integrator1/1
  Integrator1/1 -> Minus/1, MORE Vehicle distance/1
  Minus/1 -> Distance Gap/1  "Distance Gap"
  Signal Builder/1(Signal 1) -> Integrator/1

== system ACC_test_sim/Switch Force Control/Distance control ==
  reset : Inport
  Distance setpoint : Inport  Port=2
  Reference distance : Inport  Port=3
  PID Tracking : Inport  Port=4
  Constant : Constant
  Gain : Gain  Gain=-1
  PID Controller : slpidlib/PID Controller  Controller=PID  Form=Parallel  TimeDomain=Continuous-time  UseExternalTs=off  SampleTime=-1  IntegratorMethod=Forward Euler  FilterMethod=Forward Euler  ControllerParametersSource=internal  P=500  I=0  UseKiTs=off  D=1000  N=100  UseFilter=on  TunerSelectOption=Frequency Response Based  InitialConditionSource=internal  InitialConditionForIntegrator=0  InitialConditionForFilter=0  DifferentiatorICPrevScaledInput=0  ExternalReset=either  TrackingMode=on  Kt=0  LimitOutput=on  SatLimitsSource=internal  UpperSaturationLimit=5000  LowerSaturationLimit=-5000  LinearizeAsGain=on  AntiWindupMode=clamping  Kb=1  POutMin=[]  POutMax=[]  IOutMin=[]  IOutMax=[]  DOutMin=[]  DOutMax=[]  NOutMin=[]  NOutMax=[]  SumOutMin=[]  SumOutMax=[]  SaturationOutMin=[]  SaturationOutMax=[]  PParamMin=[]  PParamMax=[]  IParamMin=[]  IParamMax=[]  DParamMin=[]  DParamMax=[]  NParamMin=[]  NParamMax=[]  KbParamMin=[]  KbParamMax=[]  KtParamMin=[]  KtParamMax=[]  KbOutMin=[]  KbOutMax=[]  KtOutMin=[]  KtOutMax=[]  IntegratorOutMin=[]  IntegratorOutMax=[]  FilterOutMin=[]  FilterOutMax=[]  SumI1OutMin=[]  SumI1OutMax=[]  SumI2OutMin=[]  SumI2OutMax=[]  SumI3OutMin=[]  SumI3OutMax=[]  SumI4OutMin=[]  SumI4OutMax=[]  SumDOutMin=[]  SumDOutMax=[]  DifferentiatorOutMin=[]  DifferentiatorOutMax=[]  FilterDiffOutCoefMin=[]  FilterDiffOutCoefMax=[]  ReciprocalOutMin=[]  ReciprocalOutMax=[]  SumDenOutMin=[]  SumDenOutMax=[]  SumNumOutMin=[]  SumNumOutMax=[]  DivideOutMin=[]  DivideOutMax=[]  UdiffTsProdOutMin=[]  UdiffTsProdOutMax=[]  NTsProdOutMin=[]  NTsProdOutMax=[]  UintegralTsProdOutMin=[]  UintegralTsProdOutMax=[]  UngainTsProdOutMin=[]  UngainTsProdOutMax=[]  IntegratorContinuousStateAttributes=''  IntegratorStateMustResolveToSignalObject=off  IntegratorRTWStateStorageClass=Auto  FilterContinuousStateAttributes=''  FilterStateMustResolveToSignalObject=off  FilterRTWStateStorageClass=Auto  ParallelPVariant=InternalParameters  IdealPVariant=Disabled  IVariant=InternalParameters  DVariant=InternalParameters  IntegratorVariant=Continuous  SatVariant=Enabled  AWVariant=ContClampingParallel  PCopyVariant=Disabled  TRVariant=Enabled  FdbkBlocksVariant=Forward  IdealPFdbkVariant=Disabled  SatFdbkVariant=Disabled  DerivativeFilterVariant=ContFilter  NVariant=InternalParameters  NCopyVariant=Disabled  FilterICVariant=InternalICsFilter  IntegratorICVariant=InternalICs  ExternalResetVariant=ExternalReset  TRSumVariant=TrackingMode  SumFdbkVariant=Disabled  SumVariant=Sum_PID  TsampFilterVariant=InternalTs  TsampNgainVariant=Passthrough  TsampIntegralVariant=Passthrough  ExternalSaturationOutDataTypeStr=Inherit: Same as second input  aMode=0
  Scope : Scope
  Scope1 : Scope
  Sum1 : Sum  Inputs=|+-
  Control effort : Outport
  wires:
  Sum1/1 -> Scope1/1, PID Controller/1  "E"
  Distance setpoint/1 -> Sum1/1
  PID Controller/1 -> Gain/1  "Controller Output, Force"
  Reference distance/1 -> Sum1/2
  Gain/1 -> Scope/1, Control effort/1
  reset/1 -> PID Controller/2
  PID Tracking/1 -> PID Controller/3

== system ACC_test_sim/Switch Force Control/Speed Feedback Control ==
  Speed PID tracking : Inport
  Reference speed : Inport  Port=2
  Speed setpoint : Inport  Port=3
  Enable : EnablePort  StatesWhenEnabling=reset
  -5000 -5000 N1 : Saturate  UpperLimit=5000  LowerLimit=-5000
  Add : Sum
  F(s) : Subsystem
  PID Controller : slpidlib/PID Controller  Controller=PID  Form=Parallel  TimeDomain=Continuous-time  UseExternalTs=off  SampleTime=-1  IntegratorMethod=Forward Euler  FilterMethod=Forward Euler  ControllerParametersSource=internal  P=2000  I=50  UseKiTs=off  D=10  N=100  UseFilter=on  TunerSelectOption=Transfer Function Based (PID Tuner App)  InitialConditionSource=internal  InitialConditionForIntegrator=0  InitialConditionForFilter=0  DifferentiatorICPrevScaledInput=0  ExternalReset=none  TrackingMode=on  Kt=0  LimitOutput=on  SatLimitsSource=internal  UpperSaturationLimit=5000  LowerSaturationLimit=-5000  LinearizeAsGain=on  AntiWindupMode=none  Kb=1  POutMin=[]  POutMax=[]  IOutMin=[]  IOutMax=[]  DOutMin=[]  DOutMax=[]  NOutMin=[]  NOutMax=[]  SumOutMin=[]  SumOutMax=[]  SaturationOutMin=[]  SaturationOutMax=[]  PParamMin=[]  PParamMax=[]  IParamMin=[]  IParamMax=[]  DParamMin=[]  DParamMax=[]  NParamMin=[]  NParamMax=[]  KbParamMin=[]  KbParamMax=[]  KtParamMin=[]  KtParamMax=[]  KbOutMin=[]  KbOutMax=[]  KtOutMin=[]  KtOutMax=[]  IntegratorOutMin=[]  IntegratorOutMax=[]  FilterOutMin=[]  FilterOutMax=[]  SumI1OutMin=[]  SumI1OutMax=[]  SumI2OutMin=[]  SumI2OutMax=[]  SumI3OutMin=[]  SumI3OutMax=[]  SumI4OutMin=[]  SumI4OutMax=[]  SumDOutMin=[]  SumDOutMax=[]  DifferentiatorOutMin=[]  DifferentiatorOutMax=[]  FilterDiffOutCoefMin=[]  FilterDiffOutCoefMax=[]  ReciprocalOutMin=[]  ReciprocalOutMax=[]  SumDenOutMin=[]  SumDenOutMax=[]  SumNumOutMin=[]  SumNumOutMax=[]  DivideOutMin=[]  DivideOutMax=[]  UdiffTsProdOutMin=[]  UdiffTsProdOutMax=[]  NTsProdOutMin=[]  NTsProdOutMax=[]  UintegralTsProdOutMin=[]  UintegralTsProdOutMax=[]  UngainTsProdOutMin=[]  UngainTsProdOutMax=[]  IntegratorContinuousStateAttributes=''  IntegratorStateMustResolveToSignalObject=off  IntegratorRTWStateStorageClass=Auto  FilterContinuousStateAttributes=''  FilterStateMustResolveToSignalObject=off  FilterRTWStateStorageClass=Auto  ParallelPVariant=InternalParameters  IdealPVariant=Disabled  IVariant=InternalParameters  DVariant=InternalParameters  IntegratorVariant=Continuous  SatVariant=Enabled  AWVariant=Passthrough  PCopyVariant=Disabled  TRVariant=Enabled  FdbkBlocksVariant=Forward  IdealPFdbkVariant=Disabled  SatFdbkVariant=Disabled  DerivativeFilterVariant=ContFilter  NVariant=InternalParameters  NCopyVariant=Disabled  FilterICVariant=InternalICsFilter  IntegratorICVariant=InternalICs  ExternalResetVariant=Disabled  TRSumVariant=TrackingMode  SumFdbkVariant=Disabled  SumVariant=Sum_PID  TsampFilterVariant=InternalTs  TsampNgainVariant=Passthrough  TsampIntegralVariant=Passthrough  ExternalSaturationOutDataTypeStr=Inherit: Same as second input  aMode=0
  Scope : Scope  NumInputPorts=3
  Sum1 : Sum  Inputs=|+-
  Control effort : Outport
  wires:
  Sum1/1 -> PID Controller/1  "E"
  Speed setpoint/1 -> F(s)/1(desired speed1), Sum1/1
  -5000 -5000 N1/1 -> Control effort/1, Scope/3  "Force"
  Add/1 -> -5000 -5000 N1/1
  F(s)/1(Out1) -> Scope/1, Add/1
  PID Controller/1 -> Scope/2, Add/2  "Controller Output, Force"
  Reference speed/1 -> Sum1/2
  Speed PID tracking/1 -> PID Controller/2

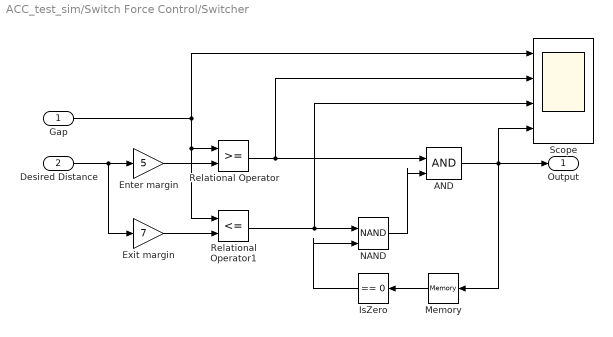
== system ACC_test_sim/Switch Force Control/Switcher ==
  Gap : Inport
  Desired Distance : Inport  Port=2
  AND : Logic  IconShape=distinctive  AllPortsSameDT=off  OutDataTypeStr=boolean
  Enter margin : Gain  Gain=5
  Exit margin : Gain  Gain=7
  IsZero : simulink/Logic and Bit Operations/Compare To Zero  relop===  OutDataTypeStr=boolean
  Memory : Memory
  NAND : Logic  Operator=NAND  IconShape=distinctive  AllPortsSameDT=off  OutDataTypeStr=boolean
  Relational Operator : RelationalOperator  OutDataTypeStr=boolean  RndMeth=Simplest  InputSameDT=off
  Relational Operator1 : RelationalOperator  Operator=<=  OutDataTypeStr=boolean  RndMeth=Simplest  InputSameDT=off
  Scope : Scope  NumInputPorts=4
  Output : Outport
  wires:
  Enter margin/1 -> Relational Operator/2
  Desired Distance/1 -> Exit margin/1, Enter margin/1
  Exit margin/1 -> Relational Operator1/2
  Relational Operator/1 -> AND/1, Scope/2
  Relational Operator1/1 -> NAND/1, Scope/3
  Memory/1 -> IsZero/1
  NAND/1 -> AND/2
  AND/1 -> Scope/4, Memory/1, Output/1
  IsZero/1 -> NAND/2
  Gap/1 -> Scope/1, Relational Operator1/1, Relational Operator/1

== system ACC_test_sim/ACC Multi MPC Speed/Sensors/Signal Builder ==
  Demux : Demux  Tag=STV Demux  Outputs=1
      settings: DisplayOption=none
  FromWs : FromWorkspace  Tag=STV FromWs  VariableName=tuvar
      SigBuilderData=|
      | common.afterFinalStr = 'Extrapolate'
      | common.sampleTime = 0
      | dataSet.timeRange = [0 100]
      | dataSet.name = 'Group 1'
      | sbobj.Groups.Name = 'Group 1'
      | sbobj.Groups.Signals.Name = 'Signal 1'
      | sbobj.Groups.Signals.XData = [0 4 35 70 100]
      | sbobj.Groups.Signals.YData = [5.55555555556 5.55555555556 5.55555555556 11.1111111111 11.1111111111]
      | sbobj.Groups.TimeRange = [0 100]
  Signal 1 : Outport  Tag=STV Outport
  wires:
  FromWs/1 -> Demux/1
  Demux/1 -> Signal 1/1

== system ACC_test_sim/ACC Multi MPC Speed/Speed Feedback Control/Feed Forward ==
  desired speed1 : Inport
  Add : Sum
  Derivative : Derivative
  Gain : Gain  Gain=b
  Gain1 : Gain  Gain=m
  Out1 : Outport
  wires:
  Gain1/1 -> Add/1
  Gain/1 -> Add/2
  Derivative/1 -> Gain1/1
  Add/1 -> Out1/1
  desired speed1/1 -> Derivative/1, Gain/1

== system ACC_test_sim/ACC Multi MPC Speed1/Sensors/Signal Builder ==
  Demux : Demux  Tag=STV Demux  Outputs=1
      settings: DisplayOption=none
  FromWs : FromWorkspace  Tag=STV FromWs  VariableName=tuvar
      SigBuilderData=|
      | common.afterFinalStr = 'Extrapolate'
      | common.sampleTime = 0
      | dataSet.timeRange = [0 100]
      | dataSet.name = 'Group 1'
      | sbobj.Groups.Name = 'Group 1'
      | sbobj.Groups.Signals.Name = 'Signal 1'
      | sbobj.Groups.Signals.XData = [0 4 35 70 100]
      | sbobj.Groups.Signals.YData = [5.55555555556 5.55555555556 5.55555555556 11.1111111111 11.1111111111]
      | sbobj.Groups.TimeRange = [0 100]
  Signal 1 : Outport  Tag=STV Outport
  wires:
  Demux/1 -> Signal 1/1
  FromWs/1 -> Demux/1

== system ACC_test_sim/ACC Multi MPC Speed1/Speed Feedback Control/Feed Forward ==
  desired speed1 : Inport
  Add : Sum
  Derivative : Derivative
  Gain : Gain  Gain=b
  Gain1 : Gain  Gain=m
  Out1 : Outport
  wires:
  desired speed1/1 -> Gain/1, Derivative/1
  Add/1 -> Out1/1
  Derivative/1 -> Gain1/1
  Gain/1 -> Add/2
  Gain1/1 -> Add/1
